simulink model "main_model"  (R2023b)
settings: Solver=FixedStepAuto  StartTime=0.0  StopTime=stopTime  RelTol=1e-3
values from neighbouring files (symbols this model uses):
  a = 6939    [Air_Drag_script.m]    (also in main.m = 6939.063; main_group24.m = 6978)
  A_BN0 = eye(3)    [main.m]
  c = 2.99792*10^8    (= 299792000)    [main.m]    (also in main_group24.m = 299792458)
  e = 0    [Air_Drag_script.m]    (also in main.m = 0.001304; main_group24.m)
  G = [gn, gm, gvali, gsvi]    [main.m]    (also in main_group24.m)
  H = [hn, hm, hvali, hsvi]    [main.m]    (also in main_group24.m)
  i = deg2rad(97.5307)    [Air_Drag_script.m]    (also in main.m; main_group24.m = deg2rad(98))
  inertia1 = Iz-Iy    (= -0.016811111)    [main.m]
  inertia2 = Ix-Iz    (= 0.033125546)    [main.m]
  inertia3 = Iy-Ix    (= -0.016314435)    [main.m]
  Inertia_matrix = [Ix 0 0; 0 Iy 0; 0 0 Iz]    [main.m]
  Inverse_inertia = inv(Inertia_matrix)    [main.m]
  m = [0.1; 0.1; 0.1]    [main.m]    (also in main_group24.m)
  MB = [4; 0.1; 0.1; 0.3]    [main.m]    (also in main_group24.m)
  mu = 3.98600433e+5    (= 398600.433)    [main.m]    (also in main_group24.m)
  n = 0.0011    [Air_Drag_script.m]    (also in main.m = sqrt(mu/a^3); main_group24.m = sqrt(mu/a^3))
  R_e = 6378    [main.m]    (also in main_group24.m)
  rho_d_MB = 0.1    [main.m]
  rho_d_SP = 0.1    [main.m]
  rho_s_MB = 0.5    [main.m]
  rho_s_SP = 0.1    [main.m]
  SP = [1; 0.3; 0.1; 0.01]    [main.m]    (also in main_group24.m = [0.25; 0.1; 0.3; 0.01])
  theta0 = deg2rad(30)    [main.m]    (also in main_group24.m = deg2rad(0))
  wx0 = deg2rad(3)    [main.m]    (also in main_group24.m)
  wy0 = deg2rad(11)    [main.m]    (also in main_group24.m)
  wz0 = deg2rad(14)    [main.m]    (also in main_group24.m)
libraries: matrix_library x8, vrlib x3, simulink_extras x1
(part 2 of 3)

== system main_model/External Torques/Solar radiation/S_B dot N_MB/If Action Subsystem ==
  NMB : Inport
  Action Port : ActionPort  ActionPortLabel=if(u1 > 0)
  Constant : Constant
  Selector : Selector  NumberOfDimensions=2  InputPortWidth=3  IndexOptions=Index vector (dialog),Index vector (dialog)  Indices=1,[1 2 3]  OutputSizes=1,1
  x : Outport
  pointer : Outport  Port=2
  wires:
  NMB/1 -> Selector/1
  Selector/1 -> x/1
  Constant/1 -> pointer/1

== system main_model/External Torques/Solar radiation/S_B dot N_MB/If Action Subsystem1 ==
  NMB : Inport
  Action Port : ActionPort  ActionPortLabel=if(u1 > 0)
  Constant : Constant
  Selector : Selector  NumberOfDimensions=2  InputPortWidth=3  IndexOptions=Index vector (dialog),Index vector (dialog)  Indices=2,[1 2 3]  OutputSizes=1,1
  y : Outport
  pointer : Outport  Port=2
  wires:
  Selector/1 -> y/1
  NMB/1 -> Selector/1
  Constant/1 -> pointer/1

== system main_model/External Torques/Solar radiation/S_B dot N_MB/If Action Subsystem2 ==
  NMB : Inport
  Action Port : ActionPort  ActionPortLabel=if(u1 > 0)
  Constant : Constant
  Selector : Selector  NumberOfDimensions=2  InputPortWidth=3  IndexOptions=Index vector (dialog),Index vector (dialog)  Indices=3,[1 2 3]  OutputSizes=1,1
  z : Outport
  pointer : Outport  Port=2
  wires:
  NMB/1 -> Selector/1
  Selector/1 -> z/1
  Constant/1 -> pointer/1

== system main_model/External Torques/Solar radiation/S_B dot N_MB/If Action Subsystem3 ==
  NMB : Inport
  Action Port : ActionPort  ActionPortLabel=else
  Constant : Constant  Value=-1
  Selector : Selector  NumberOfDimensions=2  InputPortWidth=3  IndexOptions=Index vector (dialog),Index vector (dialog)  Indices=4,[1 2 3]  OutputSizes=1,1
  -x : Outport
  pointer : Outport  Port=2
  wires:
  Selector/1 -> -x/1
  NMB/1 -> Selector/1
  Constant/1 -> pointer/1

== system main_model/External Torques/Solar radiation/S_B dot N_MB/If Action Subsystem4 ==
  NMB : Inport
  Action Port : ActionPort  ActionPortLabel=else
  Constant : Constant  Value=-1
  Selector : Selector  NumberOfDimensions=2  InputPortWidth=3  IndexOptions=Index vector (dialog),Index vector (dialog)  Indices=5,[1 2 3]  OutputSizes=1,1
  -y : Outport
  pointer : Outport  Port=2
  wires:
  NMB/1 -> Selector/1
  Selector/1 -> -y/1
  Constant/1 -> pointer/1

== system main_model/External Torques/Solar radiation/S_B dot N_MB/If Action Subsystem5 ==
  NMB : Inport
  Action Port : ActionPort  ActionPortLabel=else
  Constant : Constant  Value=-1
  Selector : Selector  NumberOfDimensions=2  InputPortWidth=3  IndexOptions=Index vector (dialog),Index vector (dialog)  Indices=6,[1 2 3]  OutputSizes=1,1
  -z : Outport
  pointer : Outport  Port=2
  wires:
  Selector/1 -> -z/1
  NMB/1 -> Selector/1
  Constant/1 -> pointer/1

== system main_model/External Torques/Solar radiation/S_B dot N_SP/If Action Subsystem ==
  N_SP : Inport
  Action Port : ActionPort  ActionPortLabel=if(u1 > 0)
  Constant : Constant
  Selector : Selector  NumberOfDimensions=2  InputPortWidth=3  IndexOptions=Index vector (dialog),Index vector (dialog)  Indices=1,[1 2 3]  OutputSizes=1,1
  true_NSP : Outport
  pointer : Outport  Port=2
  wires:
  N_SP/1 -> Selector/1
  Constant/1 -> pointer/1
  Selector/1 -> true_NSP/1

== system main_model/External Torques/Solar radiation/S_B dot N_SP/If Action Subsystem1 ==
  N_SP : Inport
  Action Port : ActionPort  ActionPortLabel=if(u1 > 0)
  Constant : Constant  Value=-1
  Selector : Selector  NumberOfDimensions=2  InputPortWidth=3  IndexOptions=Index vector (dialog),Index vector (dialog)  Indices=2,[1 2 3]  OutputSizes=1,1
  true_NSP : Outport
  pointer : Outport  Port=2
  wires:
  Selector/1 -> true_NSP/1
  Constant/1 -> pointer/1
  N_SP/1 -> Selector/1

== system main_model/External Torques/Solar radiation/Torque arm MB/creazione raggi vettore tra CM MB e centro facce illuminate della faccia che ha come normale l'asse i ==
  S_B : Inport
  MB : Inport  Port=2
  A_vect : Inport  Port=3
  pointer : Inport  Port=4
  Add2 : Sum  Inputs=+|+|+|+|+
  Demux1 : Demux  Outputs=3
  If Action Subsystem : Subsystem  TreatAsAtomicUnit=on
  If Action Subsystem1 : Subsystem  TreatAsAtomicUnit=on
  If Action Subsystem2 : Subsystem  TreatAsAtomicUnit=on
  If Action Subsystem3 : Subsystem  TreatAsAtomicUnit=on
  If Action Subsystem4 : Subsystem  TreatAsAtomicUnit=on
  If Action Subsystem5 : Subsystem  TreatAsAtomicUnit=on
  If Action Subsystem6 : Subsystem  TreatAsAtomicUnit=on
  If Action Subsystem8 : Subsystem  TreatAsAtomicUnit=on
  If1 : If  NumInputs=2  IfExpression=u1>0 & u2>0
  If2 : If  NumInputs=2  IfExpression=u1<0 & u2>0
  If3 : If  NumInputs=2  IfExpression=u1>0 & u2<0
  If4 : If  NumInputs=2  IfExpression=u1<0 & u2<0
  Merge{,1..3} (4 alike) : Merge
  Reshape1 : Reshape  OutputDimensionality=Column vector (2-D)
  Terminator1 : Terminator
  creating distance between cm MB and centro geom lato : Subsystem
  Out1 : Outport
  wires:
  [A_vect] -> If Action Subsystem2/1(Areas_vect)
  [A_vect] -> If Action Subsystem1/1(Areas_vect)
  [A_vect] -> If Action Subsystem4/1(Areas_vect)
  Add2/1 -> Out1/1
  Merge3/1 -> Add2/5  "raggio vettore centro geom lato- centro geom lato illuminato"
  If4/1 -> If Action Subsystem2/Action
  If Action Subsystem2/1(r_cface_cluce_yneg_z_neg) -> Merge3/1
  If3/1 -> If Action Subsystem1/Action
  [A_vect] -> If Action Subsystem/1(Areas_vect)
  Merge1/1 -> Add2/3  "raggio vettore centro geom lato- centro geom lato illuminato"
  If Action Subsystem4/1(r_cface_cluce_zneg_y_pos) -> Merge1/1
  Merge/1 -> Add2/2  "raggio vettore centro geom lato- centro geom lato illuminato"
  If Action Subsystem/1(r_cface_cluce_yz_pos) -> Merge/1
  If1/2 -> If Action Subsystem8/Action
  S_B/1 -> Reshape1/1
  Reshape1/1 -> Demux1/1
  Demux1/2 -> If2/2, If3/2, If4/2, If1/2  "S_B_y"
  If2/1 -> If Action Subsystem4/Action
  If1/1 -> If Action Subsystem/Action
  Demux1/3 -> If4/1, If3/1, If2/1, If1/1  "S_B_z"
  creating distance between cm MB and centro geom lato/1(Out1) -> Add2/1
  Demux1/1 -> Terminator1/1  "S_B_x"
  MB/1 -> [MB]
  [MB] -> If Action Subsystem/2(MB)
  [MB] -> If Action Subsystem4/2(MB)
  [MB] -> If Action Subsystem1/2(MB)
  [MB] -> If Action Subsystem2/2(MB)
  If Action Subsystem8/1(Out1) -> Merge/2
  If2/2 -> If Action Subsystem3/Action
  If3/2 -> If Action Subsystem5/Action
  If4/2 -> If Action Subsystem6/Action
  If Action Subsystem3/1(Out1) -> Merge1/2
  If Action Subsystem1/1(r_cface_cluce_yneg_z_pos) -> Merge2/1
  If Action Subsystem5/1(Out1) -> Merge2/2
  Merge2/1 -> Add2/4  "raggio vettore centro geom lato- centro geom lato illuminato"
  If Action Subsystem6/1(Out1) -> Merge3/2
  [MB] -> creating distance between cm MB and centro geom lato/1(MB)
  A_vect/1 -> [A_vect]
  pointer/1 -> creating distance between cm MB and centro geom lato/2(pointer)

== system main_model/External Torques/Solar radiation/Torque arm MB/creazione raggi vettore tra CM MB e centro facce illuminate della faccia che ha come normale l'asse j ==
  S_B : Inport
  MB : Inport  Port=2
  A_vect : Inport  Port=3
  pointer : Inport  Port=4
  Add2 : Sum  Inputs=+|+|+|+|+
  Demux1 : Demux  Outputs=3
  If Action Subsystem : Subsystem  TreatAsAtomicUnit=on
  If Action Subsystem1 : Subsystem  TreatAsAtomicUnit=on
  If Action Subsystem2 : Subsystem  TreatAsAtomicUnit=on
  If Action Subsystem3 : Subsystem  TreatAsAtomicUnit=on
  If Action Subsystem4 : Subsystem  TreatAsAtomicUnit=on
  If Action Subsystem5 : Subsystem  TreatAsAtomicUnit=on
  If Action Subsystem6 : Subsystem  TreatAsAtomicUnit=on
  If Action Subsystem7 : Subsystem  TreatAsAtomicUnit=on
  If1 : If  NumInputs=2  IfExpression=u1>0 & u2>0
  If2 : If  NumInputs=2  IfExpression=u1<0 & u2>0
  If3 : If  NumInputs=2  IfExpression=u1>0 & u2<0
  If4 : If  NumInputs=2  IfExpression=u1<0 & u2<0
  Merge{,1..3} (4 alike) : Merge
  Reshape1 : Reshape  OutputDimensionality=Column vector (2-D)
  Terminator1 : Terminator
  creating distance between cm MB and centro geom lato1 : Subsystem
  Out1 : Outport
  wires:
  Demux1/2 -> Terminator1/1
  creating distance between cm MB and centro geom lato1/1(Out1) -> Add2/1
  If1/1 -> If Action Subsystem/Action
  If2/1 -> If Action Subsystem1/Action
  Reshape1/1 -> Demux1/1
  S_B/1 -> Reshape1/1
  If Action Subsystem/1(r_cface_cluce_xz_pos) -> Merge/1
  Merge/1 -> Add2/2  "raggio vettore centro geom lato- centro geom lato illuminato"
  If Action Subsystem1/1(r_cface_cluce_x_pos_z_neg) -> Merge1/1
  Merge1/1 -> Add2/3  "raggio vettore centro geom lato- centro geom lato illuminato"
  [A_vect] -> If Action Subsystem/1(Areas_vect)
  Merge2/1 -> Add2/4  "raggio vettore centro geom lato- centro geom lato illuminato"
  If3/1 -> If Action Subsystem2/Action
  If Action Subsystem3/1(r_cface_cluce_x_neg_z_neg) -> Merge3/1
  If4/1 -> If Action Subsystem3/Action
  Merge3/1 -> Add2/5  "raggio vettore centro geom lato- centro geom lato illuminato"
  Add2/1 -> Out1/1
  [A_vect] -> If Action Subsystem1/1(Areas_vect)
  [A_vect] -> If Action Subsystem2/1(Areas_vect)
  [A_vect] -> If Action Subsystem3/1(Areas_vect)
  Demux1/3 -> If4/1, If3/1, If2/1, If1/1  "S_B_z"
  Demux1/1 -> If1/2, If4/2, If3/2, If2/2  "S_B_x"
  MB/1 -> [MB]
  [MB] -> If Action Subsystem/2(MB)
  [MB] -> If Action Subsystem1/2(MB)
  [MB] -> If Action Subsystem2/2(MB)
  [MB] -> If Action Subsystem3/2(MB)
  If1/2 -> If Action Subsystem5/Action
  If2/2 -> If Action Subsystem4/Action
  If3/2 -> If Action Subsystem6/Action
  If4/2 -> If Action Subsystem7/Action
  If Action Subsystem5/1(Out1) -> Merge/2
  If Action Subsystem4/1(Out1) -> Merge1/2
  If Action Subsystem2/1(r_cface_cluce_x_neg_z_pos) -> Merge2/1
  If Action Subsystem6/1(Out1) -> Merge2/2
  If Action Subsystem7/1(Out1) -> Merge3/2
  [MB] -> creating distance between cm MB and centro geom lato1/1(MB)
  A_vect/1 -> [A_vect]
  pointer/1 -> creating distance between cm MB and centro geom lato1/2(pointer)

== system main_model/External Torques/Solar radiation/Torque arm MB/creazione raggi vettore tra CM MB e centro facce illuminate della faccia che ha come normale l'asse k ==
  S_B : Inport
  MB : Inport  Port=2
  A_vect : Inport  Port=3
  pointer : Inport  Port=4
  Add2 : Sum  Inputs=+|+|+|+|+
  Demux1 : Demux  Outputs=3
  If Action Subsystem : Subsystem  TreatAsAtomicUnit=on
  If Action Subsystem1 : Subsystem  TreatAsAtomicUnit=on
  If Action Subsystem2 : Subsystem  TreatAsAtomicUnit=on
  If Action Subsystem3 : Subsystem  TreatAsAtomicUnit=on
  If Action Subsystem4 : Subsystem  TreatAsAtomicUnit=on
  If Action Subsystem5 : Subsystem  TreatAsAtomicUnit=on
  If Action Subsystem6 : Subsystem  TreatAsAtomicUnit=on
  If Action Subsystem7 : Subsystem  TreatAsAtomicUnit=on
  If1 : If  NumInputs=2  IfExpression=u1>0 & u2>0
  If2 : If  NumInputs=2  IfExpression=u1<0 & u2>0
  If3 : If  NumInputs=2  IfExpression=u1>0 & u2<0
  If4 : If  NumInputs=2  IfExpression=u1<0 & u2<0
  Merge{,1..3} (4 alike) : Merge
  Reshape1 : Reshape  OutputDimensionality=Column vector (2-D)
  Terminator1 : Terminator
  creating distance between cm MB and centro geom lato1 : Subsystem
  Out1 : Outport
  wires:
  Demux1/3 -> Terminator1/1
  Demux1/1 -> If1/1, If4/1, If3/1, If2/1  "S_B_x"
  If1/1 -> If Action Subsystem/Action
  If2/1 -> If Action Subsystem4/Action
  Demux1/2 -> If4/2, If3/2, If2/2, If1/2  "S_B_y"
  Reshape1/1 -> Demux1/1
  S_B/1 -> Reshape1/1
  If1/2 -> If Action Subsystem5/Action
  Merge/1 -> Add2/2  "raggio vettore centro geom lato- centro geom lato illuminato"
  Merge1/1 -> Add2/3  "raggio vettore centro geom lato- centro geom lato illuminato"
  [A_vect] -> If Action Subsystem/1(Areas_vect)
  Merge2/1 -> Add2/4  "raggio vettore centro geom lato- centro geom lato illuminato"
  If3/2 -> If Action Subsystem6/Action
  If Action Subsystem1/1(r_cface_cluce_xpos_y_neg) -> Merge2/1
  If3/1 -> If Action Subsystem1/Action
  If4/2 -> If Action Subsystem7/Action
  If4/1 -> If Action Subsystem2/Action
  Merge3/1 -> Add2/5  "raggio vettore centro geom lato- centro geom lato illuminato"
  Add2/1 -> Out1/1
  [A_vect] -> If Action Subsystem4/1(Areas_vect)
  [A_vect] -> If Action Subsystem1/1(Areas_vect)
  [A_vect] -> If Action Subsystem2/1(Areas_vect)
  MB/1 -> [MB]
  [MB] -> If Action Subsystem/2(MB)
  [MB] -> If Action Subsystem4/2(MB1)
  [MB] -> If Action Subsystem1/2(MB)
  [MB] -> If Action Subsystem2/2(MB1)
  If2/2 -> If Action Subsystem3/Action
  If Action Subsystem/1(r_cface_cluce_xy_pos) -> Merge/1
  If Action Subsystem5/1(Out1) -> Merge/2
  If Action Subsystem4/1(r_cface_cluce_xneg_y_pos) -> Merge1/1
  If Action Subsystem3/1(Out1) -> Merge1/2
  If Action Subsystem6/1(Out1) -> Merge2/2
  If Action Subsystem2/1(r_cface_cluce_xneg_y_neg) -> Merge3/1
  If Action Subsystem7/1(Out1) -> Merge3/2
  [MB] -> creating distance between cm MB and centro geom lato1/1(MB)
  creating distance between cm MB and centro geom lato1/1(Out1) -> Add2/1
  A_vect/1 -> [A_vect]
  pointer/1 -> creating distance between cm MB and centro geom lato1/2(pointer)

== system main_model/External Torques/Solar radiation/Torque arm SP/creazione raggi vettore tra CM SP e centro facce illuminate della faccia che ha come normale l'asse j ==
  S_B : Inport
  SP : Inport  Port=2
  A_vect : Inport  Port=3
  pointer : Inport  Port=4
  Add2 : Sum  Inputs=+|+|+|+|+
  Demux1 : Demux  Outputs=3
  If Action Subsystem : Subsystem  TreatAsAtomicUnit=on
  If Action Subsystem1 : Subsystem  TreatAsAtomicUnit=on
  If Action Subsystem2 : Subsystem  TreatAsAtomicUnit=on
  If Action Subsystem3 : Subsystem  TreatAsAtomicUnit=on
  If Action Subsystem4 : Subsystem  TreatAsAtomicUnit=on
  If Action Subsystem5 : Subsystem  TreatAsAtomicUnit=on
  If Action Subsystem6 : Subsystem  TreatAsAtomicUnit=on
  If Action Subsystem7 : Subsystem  TreatAsAtomicUnit=on
  If1 : If  NumInputs=2  IfExpression=u1>0 & u2>0
  If2 : If  NumInputs=2  IfExpression=u1<0 & u2>0
  If3 : If  NumInputs=2  IfExpression=u1>0 & u2<0
  If4 : If  NumInputs=2  IfExpression=u1<0 & u2<0
  Merge{,1..3} (4 alike) : Merge
  Reshape1 : Reshape  OutputDimensionality=Column vector (2-D)
  Terminator1 : Terminator
  creating distance between cm MB and centro geom lato1 : Subsystem
  distance : Outport
  wires:
  Demux1/2 -> Terminator1/1
  creating distance between cm MB and centro geom lato1/1(Out1) -> Add2/1
  If1/1 -> If Action Subsystem/Action
  If2/1 -> If Action Subsystem1/Action
  Reshape1/1 -> Demux1/1
  S_B/1 -> Reshape1/1
  If Action Subsystem/1(r_cface_cluce_xz_pos) -> Merge/1
  Merge/1 -> Add2/2  "raggio vettore centro geom lato- centro geom lato illuminato"
  If Action Subsystem1/1(r_cface_cluce_x_pos_z_neg) -> Merge1/1
  Merge1/1 -> Add2/3  "raggio vettore centro geom lato- centro geom lato illuminato"
  [A_vect] -> If Action Subsystem/1(Areas_vect)
  Merge2/1 -> Add2/4  "raggio vettore centro geom lato- centro geom lato illuminato"
  If3/1 -> If Action Subsystem2/Action
  If Action Subsystem3/1(r_cface_cluce_x_neg_z_neg) -> Merge3/1
  If4/1 -> If Action Subsystem3/Action
  Merge3/1 -> Add2/5  "raggio vettore centro geom lato- centro geom lato illuminato"
  Add2/1 -> distance/1
  [A_vect] -> If Action Subsystem1/1(Areas_vect)
  [A_vect] -> If Action Subsystem2/1(Areas_vect)
  [A_vect] -> If Action Subsystem3/1(Areas_vect)
  Demux1/3 -> If4/1, If3/1, If2/1, If1/1  "S_B_z"
  Demux1/1 -> If1/2, If4/2, If3/2, If2/2  "S_B_x"
  SP/1 -> [MB]
  [MB] -> If Action Subsystem/2(MB)
  [MB] -> If Action Subsystem1/2(MB)
  [MB] -> If Action Subsystem2/2(MB)
  [MB] -> If Action Subsystem3/2(MB)
  If1/2 -> If Action Subsystem5/Action
  If2/2 -> If Action Subsystem4/Action
  If3/2 -> If Action Subsystem6/Action
  If4/2 -> If Action Subsystem7/Action
  If Action Subsystem5/1(Out1) -> Merge/2
  If Action Subsystem4/1(Out1) -> Merge1/2
  If Action Subsystem2/1(r_cface_cluce_x_neg_z_pos) -> Merge2/1
  If Action Subsystem6/1(Out1) -> Merge2/2
  If Action Subsystem7/1(Out1) -> Merge3/2
  [MB] -> creating distance between cm MB and centro geom lato1/1(MB)
  A_vect/1 -> [A_vect]
  pointer/1 -> creating distance between cm MB and centro geom lato1/2(pointer)

== system main_model/External Torques/Solar radiation/Torque arm MB/creazione raggi vettore tra CM MB e centro facce illuminate della faccia che ha come normale l'asse i/If Action Subsystem ==
  Areas_vect : Inport
  MB : Inport  Port=2
  Action Port : ActionPort  ActionPortLabel=if(u1>0 & u2>0)
  Add : Sum  Inputs=+|-
  Add1 : Sum  Inputs=+|-
  Add2 : Sum
  Demux : Demux  Outputs=3
  Demux2 : Demux
  Divide : Product  Inputs=*/
  Divide1 : Product  Inputs=*/
  Gain{,1..3} (4 alike) : Gain  Gain=1/2
  Ground : Ground
  Ground1 : Ground
  Mux : Mux  Inputs=3
  Mux1 : Mux  Inputs=3
  Reshape : Reshape  OutputDimensionality=Column vector (2-D)
  Reshape2 : Reshape  OutputDimensionality=Column vector (2-D)
  Reshape3 : Reshape  OutputDimensionality=Column vector (2-D)
  Terminator{1..2,8..9} (4 alike) : Terminator
  r_cface_cluce_yz_pos : Outport
  wires:
  Demux/2 -> Terminator8/1
  Demux/3 -> Terminator9/1
  Add2/1 -> r_cface_cluce_yz_pos/1
  Reshape3/1 -> Add2/2
  Reshape2/1 -> Add2/1
  [h_MB] -> Gain2/1
  Divide1/1 -> Gain3/1
  Gain2/1 -> Add1/1
  Gain3/1 -> Add1/2
  Ground/1 -> Mux1/2, Mux1/1
  Mux1/1 -> Reshape3/1  "raggio vettore che collega il centro geom della faccia con il centro geom della faccia illuminata dal sole lungo k"
  [b_MB] -> Divide1/2
  Reshape/1 -> Demux/1
  Ground1/1 -> Mux/3, Mux/1
  Areas_vect/1 -> Reshape/1
  [h_MB] -> Divide/2
  Gain/1 -> Add/1
  [b_MB] -> Gain/1
  Gain1/1 -> Add/2
  Mux/1 -> Reshape2/1  "raggio vettore che collega il centro geom della faccia con il centro geom della faccia illuminata dal sole lungo j"
  Divide/1 -> Gain1/1
  Demux/1 -> Divide1/1, Divide/1
  Add/1 -> Mux/2
  Add1/1 -> Mux1/3
  Demux2/1 -> Terminator2/1
  Demux2/2 -> Terminator1/1
  MB/1 -> Demux2/1
  Demux2/3 -> [b_MB]
  Demux2/4 -> [h_MB]

== system main_model/External Torques/Solar radiation/Torque arm MB/creazione raggi vettore tra CM MB e centro facce illuminate della faccia che ha come normale l'asse i/If Action Subsystem1 ==
  Areas_vect : Inport
  MB : Inport  Port=2
  Action Port : ActionPort  ActionPortLabel=if(u1>0 & u2<0)
  Add : Sum  Inputs=+|-
  Add1 : Sum  Inputs=+|-
  Add2 : Sum
  Demux : Demux  Outputs=3
  Demux2 : Demux
  Divide : Product  Inputs=*/
  Divide1 : Product  Inputs=*/
  Gain{,1..3} (4 alike) : Gain  Gain=1/2
  Gain4 : Gain  Gain=-1
  Ground : Ground
  Ground1 : Ground
  Mux : Mux  Inputs=3
  Mux1 : Mux  Inputs=3
  Reshape : Reshape  OutputDimensionality=Column vector (2-D)
  Reshape2 : Reshape  OutputDimensionality=Column vector (2-D)
  Reshape3 : Reshape  OutputDimensionality=Column vector (2-D)
  Terminator{1..2,8..9} (4 alike) : Terminator
  r_cface_cluce_yneg_z_pos : Outport
  wires:
  Add1/1 -> Mux1/3
  Demux/1 -> Divide/1, Divide1/1
  Divide/1 -> Gain1/1
  Mux/1 -> Reshape2/1  "raggio vettore che collega il centro geom della faccia con il centro geom della faccia illuminata dal sole lungo -j"
  Gain1/1 -> Add/2
  [b_MB] -> Gain/1
  Gain/1 -> Add/1
  [h_MB] -> Divide/2
  Areas_vect/1 -> Reshape/1
  Ground1/1 -> Mux/1, Mux/3
  Reshape/1 -> Demux/1
  [b_MB] -> Divide1/2
  Mux1/1 -> Reshape3/1  "raggio vettore che collega il centro geom della faccia con il centro geom della faccia illuminata dal sole lungo k"
  Ground/1 -> Mux1/1, Mux1/2
  Gain3/1 -> Add1/2
  Gain2/1 -> Add1/1
  Divide1/1 -> Gain3/1
  [h_MB] -> Gain2/1
  Reshape2/1 -> Add2/1
  Reshape3/1 -> Add2/2
  Add2/1 -> r_cface_cluce_yneg_z_pos/1
  Demux/3 -> Terminator9/1
  Demux/2 -> Terminator8/1
  Add/1 -> Gain4/1
  Gain4/1 -> Mux/2
  Demux2/1 -> Terminator2/1
  Demux2/2 -> Terminator1/1
  MB/1 -> Demux2/1
  Demux2/3 -> [b_MB]
  Demux2/4 -> [h_MB]

== system main_model/External Torques/Solar radiation/Torque arm MB/creazione raggi vettore tra CM MB e centro facce illuminate della faccia che ha come normale l'asse i/If Action Subsystem2 ==
  Areas_vect : Inport
  MB : Inport  Port=2
  Action Port : ActionPort  ActionPortLabel=if(u1<0 & u2<0)
  Add : Sum  Inputs=+|-
  Add1 : Sum  Inputs=+|-
  Add2 : Sum
  Demux : Demux  Outputs=3
  Demux2 : Demux
  Divide : Product  Inputs=*/
  Divide1 : Product  Inputs=*/
  Gain{,1..3} (4 alike) : Gain  Gain=1/2
  Gain4 : Gain  Gain=-1
  Gain5 : Gain  Gain=-1
  Ground : Ground
  Ground1 : Ground
  Mux : Mux  Inputs=3
  Mux1 : Mux  Inputs=3
  Reshape : Reshape  OutputDimensionality=Column vector (2-D)
  Reshape2 : Reshape  OutputDimensionality=Column vector (2-D)
  Reshape3 : Reshape  OutputDimensionality=Column vector (2-D)
  Terminator{1..2,8..9} (4 alike) : Terminator
  r_cface_cluce_yneg_z_neg : Outport
  wires:
  Gain4/1 -> Mux/2
  Add/1 -> Gain4/1
  Demux/2 -> Terminator8/1
  Demux/3 -> Terminator9/1
  Add2/1 -> r_cface_cluce_yneg_z_neg/1
  Reshape3/1 -> Add2/2
  Reshape2/1 -> Add2/1
  [h_MB] -> Gain2/1
  Divide1/1 -> Gain3/1
  Gain2/1 -> Add1/1
  Gain3/1 -> Add1/2
  Ground/1 -> Mux1/2, Mux1/1
  Mux1/1 -> Reshape3/1  "raggio vettore che collega il centro geom della faccia con il centro geom della faccia illuminata dal sole lungo -k"
  [b_MB] -> Divide1/2
  Reshape/1 -> Demux/1
  Ground1/1 -> Mux/3, Mux/1
  Areas_vect/1 -> Reshape/1
  [h_MB] -> Divide/2
  Gain/1 -> Add/1
  [b_MB] -> Gain/1
  Gain1/1 -> Add/2
  Mux/1 -> Reshape2/1  "raggio vettore che collega il centro geom della faccia con il centro geom della faccia illuminata dal sole lungo -j"
  Divide/1 -> Gain1/1
  Demux/1 -> Divide1/1, Divide/1
  Gain5/1 -> Mux1/3
  Add1/1 -> Gain5/1
  Demux2/1 -> Terminator2/1
  Demux2/2 -> Terminator1/1
  MB/1 -> Demux2/1
  Demux2/3 -> [b_MB]
  Demux2/4 -> [h_MB]

== system main_model/External Torques/Solar radiation/Torque arm MB/creazione raggi vettore tra CM MB e centro facce illuminate della faccia che ha come normale l'asse i/If Action Subsystem3 ==
  Action Port : ActionPort  ActionPortLabel=else
  Constant : Constant  Value=[0;0;0]
  Out1 : Outport
  wires:
  Constant/1 -> Out1/1

== system main_model/External Torques/Solar radiation/Torque arm MB/creazione raggi vettore tra CM MB e centro facce illuminate della faccia che ha come normale l'asse i/If Action Subsystem4 ==
  Areas_vect : Inport
  MB : Inport  Port=2
  Action Port : ActionPort  ActionPortLabel=if(u1<0 & u2>0)
  Add : Sum  Inputs=+|-
  Add1 : Sum  Inputs=+|-
  Add2 : Sum
  Demux : Demux  Outputs=3
  Demux2 : Demux
  Divide : Product  Inputs=*/
  Divide1 : Product  Inputs=*/
  Gain{,1..3} (4 alike) : Gain  Gain=1/2
  Gain4 : Gain  Gain=-1
  Ground : Ground
  Ground1 : Ground
  Mux : Mux  Inputs=3
  Mux1 : Mux  Inputs=3
  Reshape : Reshape  OutputDimensionality=Column vector (2-D)
  Reshape2 : Reshape  OutputDimensionality=Column vector (2-D)
  Reshape3 : Reshape  OutputDimensionality=Column vector (2-D)
  Terminator{1..2,8..9} (4 alike) : Terminator
  r_cface_cluce_zneg_y_pos : Outport
  wires:
  [h_MB] -> Divide1/2
  [b_MB] -> Gain2/1
  Add1/1 -> Mux1/2
  Gain4/1 -> Mux/3
  Add/1 -> Gain4/1
  [h_MB] -> Gain/1
  [b_MB] -> Divide/2
  Divide/1 -> Gain1/1
  Mux/1 -> Reshape2/1  "raggio vettore che collega il centro geom della faccia con il centro geom della faccia illuminata dal sole lungo -k"
  Gain1/1 -> Add/2
  Gain/1 -> Add/1
  Areas_vect/1 -> Reshape/1
  Ground1/1 -> Mux/1, Mux/2
  Reshape/1 -> Demux/1
  Mux1/1 -> Reshape3/1  "raggio vettore che collega il centro geom della faccia con il centro geom della faccia illuminata dal sole lungo j"
  Ground/1 -> Mux1/3, Mux1/1
  Gain3/1 -> Add1/2
  Gain2/1 -> Add1/1
  Divide1/1 -> Gain3/1
  Reshape2/1 -> Add2/1
  Reshape3/1 -> Add2/2
  Add2/1 -> r_cface_cluce_zneg_y_pos/1
  Demux/2 -> Terminator9/1
  Demux/3 -> Terminator8/1
  Demux/1 -> Divide1/1, Divide/1
  Demux2/1 -> Terminator2/1
  Demux2/2 -> Terminator1/1
  MB/1 -> Demux2/1
  Demux2/3 -> [b_MB]
  Demux2/4 -> [h_MB]

== system main_model/External Torques/Solar radiation/Torque arm MB/creazione raggi vettore tra CM MB e centro facce illuminate della faccia che ha come normale l'asse i/If Action Subsystem5 ==
  Action Port : ActionPort  ActionPortLabel=else
  Constant : Constant  Value=[0;0;0]
  Out1 : Outport
  wires:
  Constant/1 -> Out1/1

== system main_model/External Torques/Solar radiation/Torque arm MB/creazione raggi vettore tra CM MB e centro facce illuminate della faccia che ha come normale l'asse i/If Action Subsystem6 ==
  Action Port : ActionPort  ActionPortLabel=else
  Constant : Constant  Value=[0;0;0]
  Out1 : Outport
  wires:
  Constant/1 -> Out1/1

== system main_model/External Torques/Solar radiation/Torque arm MB/creazione raggi vettore tra CM MB e centro facce illuminate della faccia che ha come normale l'asse i/If Action Subsystem8 ==
  Action Port : ActionPort  ActionPortLabel=else
  Constant : Constant  Value=[0;0;0]
  Out1 : Outport
  wires:
  Constant/1 -> Out1/1

== system main_model/External Torques/Solar radiation/Torque arm MB/creazione raggi vettore tra CM MB e centro facce illuminate della faccia che ha come normale l'asse i/creating distance between cm MB and centro geom lato ==
  MB : Inport
  pointer : Inport  Port=2
  Demux : Demux
  Ground : Ground
  Mux : Mux  Inputs=3
  Product : Product
  Reshape : Reshape  OutputDimensionality=Column vector (2-D)
  Terminator : Terminator
  Terminator1 : Terminator
  Terminator3 : Terminator
  Out1 : Outport
  wires:
  Reshape/1 -> Out1/1
  Mux/1 -> Reshape/1
  MB/1 -> Demux/1
  Demux/1 -> Terminator/1
  Demux/2 -> Terminator1/1
  Ground/1 -> Mux/3, Mux/1
  Demux/4 -> Terminator3/1
  Demux/3 -> Product/1
  Product/1 -> Mux/2
  pointer/1 -> Product/2

== system main_model/External Torques/Solar radiation/Torque arm MB/creazione raggi vettore tra CM MB e centro facce illuminate della faccia che ha come normale l'asse j/If Action Subsystem ==
  Areas_vect : Inport
  MB : Inport  Port=2
  Action Port : ActionPort  ActionPortLabel=if(u1>0 & u2>0)
  Add : Sum  Inputs=+|-
  Add1 : Sum  Inputs=+|-
  Add2 : Sum
  Demux : Demux  Outputs=3
  Demux2 : Demux
  Divide : Product  Inputs=*/
  Divide1 : Product  Inputs=*/
  Gain{,1..3} (4 alike) : Gain  Gain=1/2
  Ground : Ground
  Ground1 : Ground
  Mux : Mux  Inputs=3
  Mux1 : Mux  Inputs=3
  Reshape : Reshape  OutputDimensionality=Column vector (2-D)
  Reshape2 : Reshape  OutputDimensionality=Column vector (2-D)
  Reshape3 : Reshape  OutputDimensionality=Column vector (2-D)
  Terminator{1..2,8..9} (4 alike) : Terminator
  r_cface_cluce_xz_pos : Outport
  wires:
  Add/1 -> Mux/3
  Divide/1 -> Gain1/1
  Mux/1 -> Reshape2/1  "raggio vettore che collega il centro geom della faccia con il centro geom della faccia illuminata dal sole lungo k"
  Gain1/1 -> Add/2
  Demux/2 -> Divide1/1, Divide/1
  [h_MB] -> Gain/1
  Gain/1 -> Add/1
  [a_MB] -> Divide/2
  Areas_vect/1 -> Reshape/1
  Ground1/1 -> Mux/2, Mux/1
  Reshape/1 -> Demux/1
  Add1/1 -> Mux1/1
  [h_MB] -> Divide1/2
  Mux1/1 -> Reshape3/1  "raggio vettore che collega il centro geom della faccia con il centro geom della faccia illuminata dal sole lungo i"
  Ground/1 -> Mux1/2, Mux1/3
  Gain3/1 -> Add1/2
  Gain2/1 -> Add1/1
  Divide1/1 -> Gain3/1
  [a_MB] -> Gain2/1
  Reshape2/1 -> Add2/1
  Reshape3/1 -> Add2/2
  Add2/1 -> r_cface_cluce_xz_pos/1
  Demux/1 -> Terminator9/1
  Demux/3 -> Terminator8/1
  Demux2/1 -> Terminator2/1
  Demux2/2 -> [a_MB]
  MB/1 -> Demux2/1
  Demux2/3 -> Terminator1/1
  Demux2/4 -> [h_MB]

== system main_model/External Torques/Solar radiation/Torque arm MB/creazione raggi vettore tra CM MB e centro facce illuminate della faccia che ha come normale l'asse j/If Action Subsystem1 ==
  Areas_vect : Inport
  MB : Inport  Port=2
  Action Port : ActionPort  ActionPortLabel=if(u1<0 & u2>0)
  Add : Sum  Inputs=+|-
  Add1 : Sum  Inputs=+|-
  Add2 : Sum
  Demux : Demux  Outputs=3
  Demux2 : Demux
  Divide : Product  Inputs=*/
  Divide1 : Product  Inputs=*/
  Gain{,1..3} (4 alike) : Gain  Gain=1/2
  Gain4 : Gain  Gain=-1
  Ground : Ground
  Ground1 : Ground
  Mux : Mux  Inputs=3
  Mux1 : Mux  Inputs=3
  Reshape : Reshape  OutputDimensionality=Column vector (2-D)
  Reshape2 : Reshape  OutputDimensionality=Column vector (2-D)
  Reshape3 : Reshape  OutputDimensionality=Column vector (2-D)
  Terminator{1..2,8..9} (4 alike) : Terminator
  r_cface_cluce_x_pos_z_neg : Outport
  wires:
  Demux/3 -> Terminator8/1
  Demux/1 -> Terminator9/1
  Add2/1 -> r_cface_cluce_x_pos_z_neg/1
  Reshape3/1 -> Add2/2
  Reshape2/1 -> Add2/1
  [a_MB] -> Gain2/1
  Divide1/1 -> Gain3/1
  Gain2/1 -> Add1/1
  Gain3/1 -> Add1/2
  Ground/1 -> Mux1/3, Mux1/2
  Mux1/1 -> Reshape3/1  "raggio vettore che collega il centro geom della faccia con il centro geom della faccia illuminata dal sole lungo i"
  [h_MB] -> Divide1/2
  Add1/1 -> Mux1/1
  Reshape/1 -> Demux/1
  Ground1/1 -> Mux/1, Mux/2
  Areas_vect/1 -> Reshape/1
  [a_MB] -> Divide/2
  Gain/1 -> Add/1
  [h_MB] -> Gain/1
  Demux/2 -> Divide/1, Divide1/1
  Gain1/1 -> Add/2
  Mux/1 -> Reshape2/1  "raggio vettore che collega il centro geom della faccia con il centro geom della faccia illuminata dal sole lungo -k"
  Divide/1 -> Gain1/1
  Add/1 -> Gain4/1
  Gain4/1 -> Mux/3
  Demux2/1 -> Terminator2/1
  Demux2/2 -> [a_MB]
  MB/1 -> Demux2/1
  Demux2/3 -> Terminator1/1
  Demux2/4 -> [h_MB]

== system main_model/External Torques/Solar radiation/Torque arm MB/creazione raggi vettore tra CM MB e centro facce illuminate della faccia che ha come normale l'asse j/If Action Subsystem2 ==
  Areas_vect : Inport
  MB : Inport  Port=2
  Action Port : ActionPort  ActionPortLabel=if(u1>0 & u2<0)
  Add : Sum  Inputs=+|-
  Add1 : Sum  Inputs=+|-
  Add2 : Sum
  Demux : Demux  Outputs=3
  Demux2 : Demux
  Divide : Product  Inputs=*/
  Divide1 : Product  Inputs=*/
  Gain{,1..3} (4 alike) : Gain  Gain=1/2
  Gain4 : Gain  Gain=-1
  Ground : Ground
  Ground1 : Ground
  Mux : Mux  Inputs=3
  Mux1 : Mux  Inputs=3
  Reshape : Reshape  OutputDimensionality=Column vector (2-D)
  Reshape2 : Reshape  OutputDimensionality=Column vector (2-D)
  Reshape3 : Reshape  OutputDimensionality=Column vector (2-D)
  Terminator{1..2,8..9} (4 alike) : Terminator
  r_cface_cluce_x_neg_z_pos : Outport
  wires:
  Add/1 -> Mux/3
  Divide/1 -> Gain1/1
  Mux/1 -> Reshape2/1  "raggio vettore che collega il centro geom della faccia con il centro geom della faccia illuminata dal sole lungo k"
  Gain1/1 -> Add/2
  Demux/2 -> Divide1/1, Divide/1
  [h_MB] -> Gain/1
  Gain/1 -> Add/1
  [a_MB] -> Divide/2
  Areas_vect/1 -> Reshape/1
  Ground1/1 -> Mux/2, Mux/1
  Reshape/1 -> Demux/1
  [h_MB] -> Divide1/2
  Mux1/1 -> Reshape3/1  "raggio vettore che collega il centro geom della faccia con il centro geom della faccia illuminata dal sole lungo -i"
  Ground/1 -> Mux1/2, Mux1/3
  Gain3/1 -> Add1/2
  Gain2/1 -> Add1/1
  Divide1/1 -> Gain3/1
  [a_MB] -> Gain2/1
  Reshape2/1 -> Add2/1
  Reshape3/1 -> Add2/2
  Add2/1 -> r_cface_cluce_x_neg_z_pos/1
  Demux/1 -> Terminator9/1
  Demux/3 -> Terminator8/1
  Gain4/1 -> Mux1/1
  Add1/1 -> Gain4/1
  Demux2/1 -> Terminator2/1
  Demux2/2 -> [a_MB]
  MB/1 -> Demux2/1
  Demux2/3 -> Terminator1/1
  Demux2/4 -> [h_MB]

== system main_model/External Torques/Solar radiation/Torque arm MB/creazione raggi vettore tra CM MB e centro facce illuminate della faccia che ha come normale l'asse j/If Action Subsystem3 ==
  Areas_vect : Inport
  MB : Inport  Port=2
  Action Port : ActionPort  ActionPortLabel=if(u1<0 & u2<0)
  Add : Sum  Inputs=+|-
  Add1 : Sum  Inputs=+|-
  Add2 : Sum
  Demux : Demux  Outputs=3
  Demux2 : Demux
  Divide : Product  Inputs=*/
  Divide1 : Product  Inputs=*/
  Gain{,1..3} (4 alike) : Gain  Gain=1/2
  Gain4 : Gain  Gain=-1
  Gain5 : Gain  Gain=-1
  Ground : Ground
  Ground1 : Ground
  Mux : Mux  Inputs=3
  Mux1 : Mux  Inputs=3
  Reshape : Reshape  OutputDimensionality=Column vector (2-D)
  Reshape2 : Reshape  OutputDimensionality=Column vector (2-D)
  Reshape3 : Reshape  OutputDimensionality=Column vector (2-D)
  Terminator{1..2,8..9} (4 alike) : Terminator
  r_cface_cluce_x_neg_z_neg : Outport
  wires:
  Add1/1 -> Gain4/1
  Gain4/1 -> Mux1/1
  Demux/3 -> Terminator8/1
  Demux/1 -> Terminator9/1
  Add2/1 -> r_cface_cluce_x_neg_z_neg/1
  Reshape3/1 -> Add2/2
  Reshape2/1 -> Add2/1
  [a_MB] -> Gain2/1
  Divide1/1 -> Gain3/1
  Gain2/1 -> Add1/1
  Gain3/1 -> Add1/2
  Ground/1 -> Mux1/3, Mux1/2
  Mux1/1 -> Reshape3/1  "raggio vettore che collega il centro geom della faccia con il centro geom della faccia illuminata dal sole lungo -i"
  [h_MB] -> Divide1/2
  Reshape/1 -> Demux/1
  Ground1/1 -> Mux/1, Mux/2
  Areas_vect/1 -> Reshape/1
  [a_MB] -> Divide/2
  Gain/1 -> Add/1
  [h_MB] -> Gain/1
  Demux/2 -> Divide/1, Divide1/1
  Gain1/1 -> Add/2
  Mux/1 -> Reshape2/1  "raggio vettore che collega il centro geom della faccia con il centro geom della faccia illuminata dal sole lungo -k"
  Divide/1 -> Gain1/1
  Add/1 -> Gain5/1
  Gain5/1 -> Mux/3
  Demux2/1 -> Terminator2/1
  Demux2/2 -> [a_MB]
  MB/1 -> Demux2/1
  Demux2/3 -> Terminator1/1
  Demux2/4 -> [h_MB]

== system main_model/External Torques/Solar radiation/Torque arm MB/creazione raggi vettore tra CM MB e centro facce illuminate della faccia che ha come normale l'asse j/If Action Subsystem4 ==
  Action Port : ActionPort  ActionPortLabel=else
  Constant : Constant  Value=[0;0;0]
  Out1 : Outport
  wires:
  Constant/1 -> Out1/1

== system main_model/External Torques/Solar radiation/Torque arm MB/creazione raggi vettore tra CM MB e centro facce illuminate della faccia che ha come normale l'asse j/If Action Subsystem5 ==
  Action Port : ActionPort  ActionPortLabel=else
  Constant : Constant  Value=[0;0;0]
  Out1 : Outport
  wires:
  Constant/1 -> Out1/1

== system main_model/External Torques/Solar radiation/Torque arm MB/creazione raggi vettore tra CM MB e centro facce illuminate della faccia che ha come normale l'asse j/If Action Subsystem6 ==
  Action Port : ActionPort  ActionPortLabel=else
  Constant : Constant  Value=[0;0;0]
  Out1 : Outport
  wires:
  Constant/1 -> Out1/1

== system main_model/External Torques/Solar radiation/Torque arm MB/creazione raggi vettore tra CM MB e centro facce illuminate della faccia che ha come normale l'asse j/If Action Subsystem7 ==
  Action Port : ActionPort  ActionPortLabel=else
  Constant : Constant  Value=[0;0;0]
  Out1 : Outport
  wires:
  Constant/1 -> Out1/1

== system main_model/External Torques/Solar radiation/Torque arm MB/creazione raggi vettore tra CM MB e centro facce illuminate della faccia che ha come normale l'asse j/creating distance between cm MB and centro geom lato1 ==
  MB : Inport
  pointer : Inport  Port=2
  Demux : Demux
  Ground : Ground
  Mux : Mux  Inputs=3
  Product : Product
  Reshape : Reshape  OutputDimensionality=Column vector (2-D)
  Terminator : Terminator
  Terminator1 : Terminator
  Terminator2 : Terminator
  Out1 : Outport
  wires:
  Reshape/1 -> Out1/1
  Mux/1 -> Reshape/1
  MB/1 -> Demux/1
  Demux/1 -> Terminator/1
  Demux/2 -> Terminator1/1
  Demux/3 -> Terminator2/1
  Ground/1 -> Mux/2, Mux/1
  Demux/4 -> Product/1
  pointer/1 -> Product/2
  Product/1 -> Mux/3

== system main_model/External Torques/Solar radiation/Torque arm MB/creazione raggi vettore tra CM MB e centro facce illuminate della faccia che ha come normale l'asse k/If Action Subsystem ==
  Areas_vect : Inport
  MB : Inport  Port=2
  Action Port : ActionPort  ActionPortLabel=if(u1>0 & u2>0)
  Add : Sum  Inputs=+|-
  Add1 : Sum  Inputs=+|-
  Add2 : Sum
  Demux : Demux  Outputs=3
  Demux1 : Demux  Outputs=3
  Demux2 : Demux
  Divide : Product  Inputs=*/
  Divide1 : Product  Inputs=*/
  Gain{,1..3} (4 alike) : Gain  Gain=1/2
  Ground : Ground
  Ground1 : Ground
  Mux : Mux  Inputs=3
  Mux1 : Mux  Inputs=3
  Reshape{,1..3} (4 alike) : Reshape  OutputDimensionality=Column vector (2-D)
  Terminator{,1..3,8..9} (6 alike) : Terminator
  r_cface_cluce_xy_pos : Outport
  wires:
  Add/1 -> Mux/2
  Divide/1 -> Gain1/1
  Mux/1 -> Reshape2/1  "raggio vettore che collega il centro geom della faccia con il centro geom della faccia illuminata dal sole lungo j"
  Gain1/1 -> Add/2
  Demux/3 -> Divide/1
  [b_MB] -> Gain/1
  Gain/1 -> Add/1
  [a_MB] -> Divide/2
  Areas_vect/1 -> Reshape/1, Reshape1/1
  Ground1/1 -> Mux/1, Mux/3
  Reshape/1 -> Demux/1
  Add1/1 -> Mux1/1
  [b_MB] -> Divide1/2
  Mux1/1 -> Reshape3/1  "raggio vettore che collega il centro geom della faccia con il centro geom della faccia illuminata dal sole lungo x"
  Ground/1 -> Mux1/2, Mux1/3
  Demux1/3 -> Divide1/1
  Gain3/1 -> Add1/2
  Gain2/1 -> Add1/1
  Reshape1/1 -> Demux1/1
  Divide1/1 -> Gain3/1
  [a_MB] -> Gain2/1
  Reshape2/1 -> Add2/1
  Reshape3/1 -> Add2/2
  Add2/1 -> r_cface_cluce_xy_pos/1
  Demux1/1 -> Terminator/1
  Demux1/2 -> Terminator1/1
  Demux/1 -> Terminator9/1
  Demux/2 -> Terminator8/1
  MB/1 -> Demux2/1
  Demux2/1 -> Terminator2/1
  Demux2/2 -> [a_MB]
  Demux2/3 -> [b_MB]
  Demux2/4 -> Terminator3/1

== system main_model/External Torques/Solar radiation/Torque arm MB/creazione raggi vettore tra CM MB e centro facce illuminate della faccia che ha come normale l'asse k/If Action Subsystem1 ==
  Areas_vect : Inport
  MB : Inport  Port=2
  Action Port : ActionPort  ActionPortLabel=if(u1>0 & u2<0)
  Add : Sum  Inputs=+|-
  Add1 : Sum  Inputs=+|-
  Add2 : Sum
  Demux : Demux  Outputs=3
  Demux1 : Demux  Outputs=3
  Demux2 : Demux
  Divide : Product  Inputs=*/
  Divide1 : Product  Inputs=*/
  Gain{,1..3} (4 alike) : Gain  Gain=1/2
  Gain4 : Gain  Gain=-1
  Ground : Ground
  Ground1 : Ground
  Mux : Mux  Inputs=3
  Mux1 : Mux  Inputs=3
  Reshape{,1..3} (4 alike) : Reshape  OutputDimensionality=Column vector (2-D)
  Terminator{,1..3,8..9} (6 alike) : Terminator
  r_cface_cluce_xpos_y_neg : Outport
  wires:
  Add/1 -> Gain4/1
  Divide/1 -> Gain1/1
  Mux/1 -> Reshape2/1  "raggio vettore che collega il centro geom della faccia con il centro geom della faccia illuminata dal sole lungo -j"
  Gain1/1 -> Add/2
  Demux/3 -> Divide/1
  Gain/1 -> Add/1
  Areas_vect/1 -> Reshape/1, Reshape1/1
  Ground1/1 -> Mux/1, Mux/3
  Reshape/1 -> Demux/1
  Mux1/1 -> Reshape3/1  "raggio vettore che collega il centro geom della faccia con il centro geom della faccia illuminata dal sole lungo i"
  Ground/1 -> Mux1/2, Mux1/3
  Demux1/3 -> Divide1/1
  Gain3/1 -> Add1/2
  Gain2/1 -> Add1/1
  Reshape1/1 -> Demux1/1
  Divide1/1 -> Gain3/1
  Reshape2/1 -> Add2/1
  Reshape3/1 -> Add2/2
  Add2/1 -> r_cface_cluce_xpos_y_neg/1
  Demux1/1 -> Terminator/1
  Demux1/2 -> Terminator1/1
  Demux/1 -> Terminator9/1
  Demux/2 -> Terminator8/1
  Gain4/1 -> Mux/2
  [a_MB] -> Divide/2
  [b_MB] -> Gain/1
  Add1/1 -> Mux1/1
  [b_MB] -> Divide1/2
  [a_MB] -> Gain2/1
  Demux2/1 -> Terminator2/1
  Demux2/2 -> [a_MB]
  MB/1 -> Demux2/1
  Demux2/3 -> [b_MB]
  Demux2/4 -> Terminator3/1

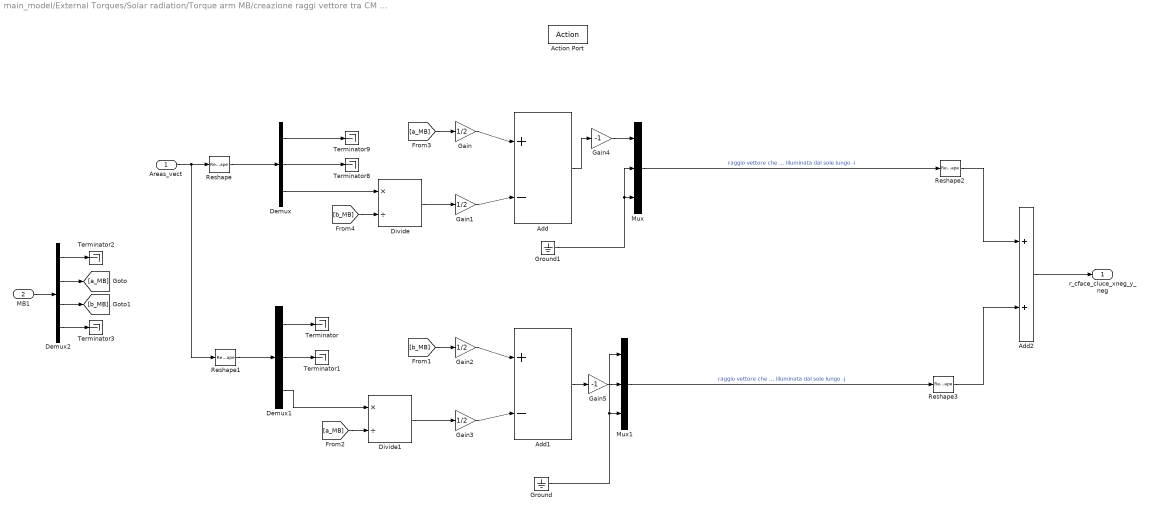
== system main_model/External Torques/Solar radiation/Torque arm MB/creazione raggi vettore tra CM MB e centro facce illuminate della faccia che ha come normale l'asse k/If Action Subsystem2 ==
  Areas_vect : Inport
  MB1 : Inport  Port=2
  Action Port : ActionPort  ActionPortLabel=if(u1<0 & u2<0)
  Add : Sum  Inputs=+|-
  Add1 : Sum  Inputs=+|-
  Add2 : Sum
  Demux : Demux  Outputs=3
  Demux1 : Demux  Outputs=3
  Demux2 : Demux
  Divide : Product  Inputs=*/
  Divide1 : Product  Inputs=*/
  Gain{,1..3} (4 alike) : Gain  Gain=1/2
  Gain4 : Gain  Gain=-1
  Gain5 : Gain  Gain=-1
  Ground : Ground
  Ground1 : Ground
  Mux : Mux  Inputs=3
  Mux1 : Mux  Inputs=3
  Reshape{,1..3} (4 alike) : Reshape  OutputDimensionality=Column vector (2-D)
  Terminator{,1..3,8..9} (6 alike) : Terminator
  r_cface_cluce_xneg_y_neg : Outport
  wires:
  [a_MB] -> Divide1/2
  [b_MB] -> Gain2/1
  Add1/1 -> Gain5/1
  Gain4/1 -> Mux/1
  Add/1 -> Gain4/1
  [a_MB] -> Gain/1
  [b_MB] -> Divide/2
  Divide/1 -> Gain1/1
  Mux/1 -> Reshape2/1  "raggio vettore che collega il centro geom della faccia con il centro geom della faccia illuminata dal sole lungo -i"
  Gain1/1 -> Add/2
  Demux/3 -> Divide/1
  Gain/1 -> Add/1
  Areas_vect/1 -> Reshape/1, Reshape1/1
  Ground1/1 -> Mux/3, Mux/2
  Reshape/1 -> Demux/1
  Mux1/1 -> Reshape3/1  "raggio vettore che collega il centro geom della faccia con il centro geom della faccia illuminata dal sole lungo -j"
  Ground/1 -> Mux1/3, Mux1/1
  Demux1/3 -> Divide1/1
  Gain3/1 -> Add1/2
  Gain2/1 -> Add1/1
  Reshape1/1 -> Demux1/1
  Divide1/1 -> Gain3/1
  Reshape2/1 -> Add2/1
  Reshape3/1 -> Add2/2
  Add2/1 -> r_cface_cluce_xneg_y_neg/1
  Demux1/1 -> Terminator/1
  Demux1/2 -> Terminator1/1
  Demux/1 -> Terminator9/1
  Demux/2 -> Terminator8/1
  Gain5/1 -> Mux1/2
  Demux2/1 -> Terminator2/1
  Demux2/2 -> [a_MB]
  MB1/1 -> Demux2/1
  Demux2/3 -> [b_MB]
  Demux2/4 -> Terminator3/1

== system main_model/External Torques/Solar radiation/Torque arm MB/creazione raggi vettore tra CM MB e centro facce illuminate della faccia che ha come normale l'asse k/If Action Subsystem3 ==
  Action Port : ActionPort  ActionPortLabel=else
  Constant : Constant  Value=[0;0;0]
  Out1 : Outport
  wires:
  Constant/1 -> Out1/1

== system main_model/External Torques/Solar radiation/Torque arm MB/creazione raggi vettore tra CM MB e centro facce illuminate della faccia che ha come normale l'asse k/If Action Subsystem4 ==
  Areas_vect : Inport
  MB1 : Inport  Port=2
  Action Port : ActionPort  ActionPortLabel=if(u1<0 & u2>0)
  Add : Sum  Inputs=+|-
  Add1 : Sum  Inputs=+|-
  Add2 : Sum
  Demux : Demux  Outputs=3
  Demux1 : Demux  Outputs=3
  Demux2 : Demux
  Divide : Product  Inputs=*/
  Divide1 : Product  Inputs=*/
  Gain{,1..3} (4 alike) : Gain  Gain=1/2
  Gain4 : Gain  Gain=-1
  Ground : Ground
  Ground1 : Ground
  Mux : Mux  Inputs=3
  Mux1 : Mux  Inputs=3
  Reshape{,1..3} (4 alike) : Reshape  OutputDimensionality=Column vector (2-D)
  Terminator{,1..3,8..9} (6 alike) : Terminator
  r_cface_cluce_xneg_y_pos : Outport
  wires:
  Demux/2 -> Terminator8/1
  Demux/1 -> Terminator9/1
  Demux1/2 -> Terminator1/1
  Demux1/1 -> Terminator/1
  Add2/1 -> r_cface_cluce_xneg_y_pos/1
  Reshape3/1 -> Add2/2
  Reshape2/1 -> Add2/1
  Divide1/1 -> Gain3/1
  Reshape1/1 -> Demux1/1
  Gain2/1 -> Add1/1
  Gain3/1 -> Add1/2
  Demux1/3 -> Divide1/1
  Ground/1 -> Mux1/1, Mux1/3
  Mux1/1 -> Reshape3/1  "raggio vettore che collega il centro geom della faccia con il centro geom della faccia illuminata dal sole lungo j"
  Reshape/1 -> Demux/1
  Ground1/1 -> Mux/2, Mux/3
  Areas_vect/1 -> Reshape1/1, Reshape/1
  Gain/1 -> Add/1
  Demux/3 -> Divide/1
  Gain1/1 -> Add/2
  Mux/1 -> Reshape2/1  "raggio vettore che collega il centro geom della faccia con il centro geom della faccia illuminata dal sole lungo -i"
  Divide/1 -> Gain1/1
  [b_MB] -> Divide/2
  [a_MB] -> Gain/1
  Add/1 -> Gain4/1
  Gain4/1 -> Mux/1
  Add1/1 -> Mux1/2
  [b_MB] -> Gain2/1
  [a_MB] -> Divide1/2
  Demux2/1 -> Terminator2/1
  Demux2/2 -> [a_MB]
  MB1/1 -> Demux2/1
  Demux2/3 -> [b_MB]
  Demux2/4 -> Terminator3/1

== system main_model/External Torques/Solar radiation/Torque arm MB/creazione raggi vettore tra CM MB e centro facce illuminate della faccia che ha come normale l'asse k/If Action Subsystem5 ==
  Action Port : ActionPort  ActionPortLabel=else
  Constant : Constant  Value=[0;0;0]
  Out1 : Outport
  wires:
  Constant/1 -> Out1/1

== system main_model/External Torques/Solar radiation/Torque arm MB/creazione raggi vettore tra CM MB e centro facce illuminate della faccia che ha come normale l'asse k/If Action Subsystem6 ==
  Action Port : ActionPort  ActionPortLabel=else
  Constant : Constant  Value=[0;0;0]
  Out1 : Outport
  wires:
  Constant/1 -> Out1/1

== system main_model/External Torques/Solar radiation/Torque arm MB/creazione raggi vettore tra CM MB e centro facce illuminate della faccia che ha come normale l'asse k/If Action Subsystem7 ==
  Action Port : ActionPort  ActionPortLabel=else
  Constant : Constant  Value=[0;0;0]
  Out1 : Outport
  wires:
  Constant/1 -> Out1/1

== system main_model/External Torques/Solar radiation/Torque arm MB/creazione raggi vettore tra CM MB e centro facce illuminate della faccia che ha come normale l'asse k/creating distance between cm MB and centro geom lato1 ==
  MB : Inport
  pointer : Inport  Port=2
  Demux : Demux
  Ground : Ground
  Mux : Mux  Inputs=3
  Product : Product
  Reshape : Reshape  OutputDimensionality=Column vector (2-D)
  Terminator : Terminator
  Terminator2 : Terminator
  Terminator3 : Terminator
  Out1 : Outport
  wires:
  Reshape/1 -> Out1/1
  Mux/1 -> Reshape/1
  MB/1 -> Demux/1
  Demux/1 -> Terminator/1
  Demux/3 -> Terminator2/1
  Ground/1 -> Mux/3, Mux/2
  Demux/4 -> Terminator3/1
  Product/1 -> Mux/1
  pointer/1 -> Product/2
  Demux/2 -> Product/1

== system main_model/External Torques/Solar radiation/Torque arm SP/creazione raggi vettore tra CM SP e centro facce illuminate della faccia che ha come normale l'asse j/If Action Subsystem ==
  Areas_vect : Inport
  MB : Inport  Port=2
  Action Port : ActionPort  ActionPortLabel=if(u1>0 & u2>0)
  Add : Sum  Inputs=+|-
  Add1 : Sum  Inputs=+|-
  Add2 : Sum
  Demux2 : Demux
  Divide : Product  Inputs=*/
  Divide1 : Product  Inputs=*/
  Gain{,1..3} (4 alike) : Gain  Gain=1/2
  Ground : Ground
  Ground1 : Ground
  Mux : Mux  Inputs=3
  Mux1 : Mux  Inputs=3
  Reshape2 : Reshape  OutputDimensionality=Column vector (2-D)
  Reshape3 : Reshape  OutputDimensionality=Column vector (2-D)
  Terminator1 : Terminator
  Terminator2 : Terminator
  r_cface_cluce_xz_pos : Outport
  wires:
  Add/1 -> Mux/1
  Divide/1 -> Gain1/1
  Mux/1 -> Reshape2/1  "raggio vettore che collega il centro geom della faccia con il centro geom della faccia illuminata dal sole lungo i"
  Gain1/1 -> Add/2
  Areas_vect/1 -> Divide1/1, Divide/1
  [b_MB] -> Gain/1
  Gain/1 -> Add/1
  [a_MB] -> Divide/2
  Ground1/1 -> Mux/2, Mux/3
  Add1/1 -> Mux1/3
  [b_MB] -> Divide1/2
  Mux1/1 -> Reshape3/1  "raggio vettore che collega il centro geom della faccia con il centro geom della faccia illuminata dal sole lungo k"
  Ground/1 -> Mux1/1, Mux1/2
  Gain3/1 -> Add1/2
  Gain2/1 -> Add1/1
  Divide1/1 -> Gain3/1
  [a_MB] -> Gain2/1
  Reshape2/1 -> Add2/1
  Reshape3/1 -> Add2/2
  Add2/1 -> r_cface_cluce_xz_pos/1
  Demux2/1 -> Terminator2/1
  Demux2/2 -> [a_MB]
  MB/1 -> Demux2/1
  Demux2/3 -> [b_MB]
  Demux2/4 -> Terminator1/1

== system main_model/External Torques/Solar radiation/Torque arm SP/creazione raggi vettore tra CM SP e centro facce illuminate della faccia che ha come normale l'asse j/If Action Subsystem1 ==
  Areas_vect : Inport
  MB : Inport  Port=2
  Action Port : ActionPort  ActionPortLabel=if(u1<0 & u2>0)
  Add : Sum  Inputs=+|-
  Add1 : Sum  Inputs=+|-
  Add2 : Sum
  Demux2 : Demux
  Divide : Product  Inputs=*/
  Divide1 : Product  Inputs=*/
  Gain{,1..3} (4 alike) : Gain  Gain=1/2
  Gain4 : Gain  Gain=-1
  Ground : Ground
  Ground1 : Ground
  Mux : Mux  Inputs=3
  Mux1 : Mux  Inputs=3
  Reshape2 : Reshape  OutputDimensionality=Column vector (2-D)
  Reshape3 : Reshape  OutputDimensionality=Column vector (2-D)
  Terminator1 : Terminator
  Terminator2 : Terminator
  r_cface_cluce_x_pos_z_neg : Outport
  wires:
  Add2/1 -> r_cface_cluce_x_pos_z_neg/1
  Reshape3/1 -> Add2/2
  Reshape2/1 -> Add2/1
  [b_MB] -> Gain2/1
  Divide1/1 -> Gain3/1
  Gain2/1 -> Add1/1
  Gain3/1 -> Add1/2
  Ground/1 -> Mux1/3, Mux1/2
  Mux1/1 -> Reshape3/1  "raggio vettore che collega il centro geom della faccia con il centro geom della faccia illuminata dal sole lungo i"
  [a_MB] -> Divide1/2
  Add1/1 -> Mux1/1
  Ground1/1 -> Mux/1, Mux/2
  [b_MB] -> Divide/2
  Gain/1 -> Add/1
  [a_MB] -> Gain/1
  Areas_vect/1 -> Divide/1, Divide1/1
  Gain1/1 -> Add/2
  Mux/1 -> Reshape2/1  "raggio vettore che collega il centro geom della faccia con il centro geom della faccia illuminata dal sole lungo -k"
  Divide/1 -> Gain1/1
  Add/1 -> Gain4/1
  Gain4/1 -> Mux/3
  Demux2/1 -> Terminator2/1
  Demux2/2 -> [a_MB]
  MB/1 -> Demux2/1
  Demux2/3 -> [b_MB]
  Demux2/4 -> Terminator1/1
